simulink model "dcmtr_cl_init"  (R2024a)
settings: Solver=ode15s  StartTime=0.0  StopTime=10  RelTol=1e-3
PostLoadFcn:
  | load('dcmtr_params.mat');
libraries: slpidlib x1
settings Model: Creator=smuckati  LastModifiedBy=smuckati
settings DebuggingCC: ParameterPrecisionLossMsg=none  UnconnectedInputMsg=warning  UnconnectedOutputMsg=warning  UnconnectedLineMsg=warning
settings ModelReferenceCC: EnableRefExpFcnMdlSchedulingChecks=on
settings RTWCC: GPUComputeCapability=3.5  DLArmComputeVersion=19.05

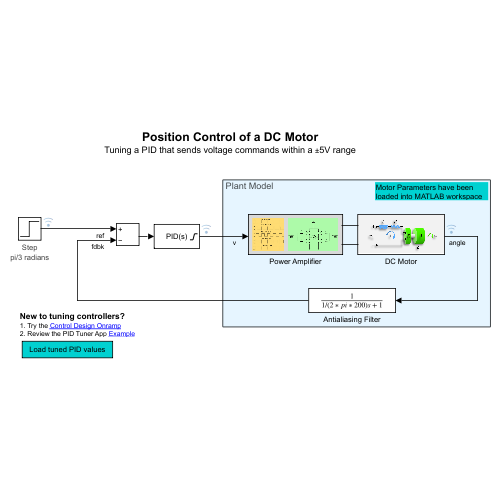
[thumbnail: Simulink's stored preview of the top-level diagram]
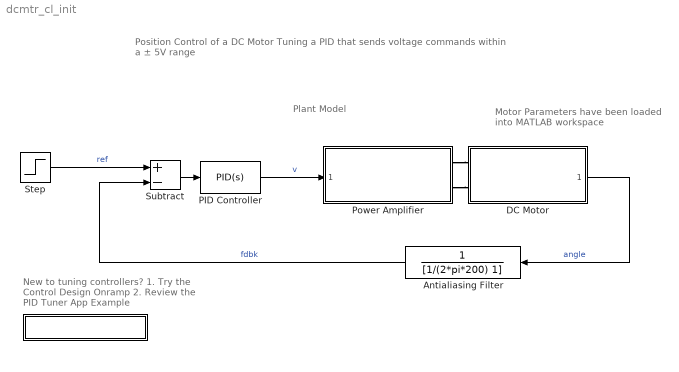
== system dcmtr_cl_init ==
  note: Motor Parameters have been loaded into MATLAB workspace
  note: Position Control of a DC Motor
      | Tuning a PID that sends voltage commands within a ± 5V range
  note: Plant Model
  note: New to tuning controllers?
      | 1. Try the Control Design Onramp
      | 2. Review the PID Tuner App Example
  "   " : Subsystem
      settings: OpenFcn=|
      | load('dcmtr_params.mat')
      | PVal = get_param('dcmtr_cl_init/PID Controller', 'P');
      | 
      | if str2num(PVal) == 1
      | set_param('dcmtr_cl_init/PID Controller', 'P', '80')
      | set_param('dcmtr_cl_init/PID Controller', 'I', '60')
      | set_param('dcmtr_cl_init/PID Controller', 'D', '-2.214')
      | set_param('dcmtr_cl_init/PID Controller', 'N', '7')
      | set_param(gcs,'SimulationCommand','update');
      | msgbox('Tuned parameters loaded to PID block')
      | end
      | 
      | if str2num(PVal) == 80
      | set_param('dcmtr_cl_init/PID Controller', 'P', '1')
      | set_param('dcmtr_cl_init/PID Controller', 'I', '1')
      | set_param('dcmtr_cl_init/PID Controller', 'D', '0')
      | set_param('dcmtr_cl_init/PID Controller', 'N', '100')
      | set_param(gcs,'SimulationCommand','update');
      | msgbox('Initial parameter values loaded to PID Block')
      | end
      mask Display:
      | PVal = get_param('dcmtr_cl_init/PID Controller', 'P');
      | 
      | if str2num(PVal) == 80
      | disp('Load initial PID values')
      | end
      | 
      | if str2num(PVal) == 1
      | disp('Load tuned PID values')
      | end
  Antialiasing Filter : TransferFcn  Denominator=[1/(2*pi*200) 1]
  DC Motor : Subsystem  ReferencedSubsystem=dcmtr
  PID Controller : slpidlib/PID Controller  Controller=PID  Form=Parallel  TimeDomain=Continuous-time  UseExternalTs=off  SampleTime=-1  IntegratorMethod=Forward Euler  FilterMethod=Forward Euler  ControllerParametersSource=internal  P=1  I=1  UseKiTs=off  D=0  UseExternalDerivativeSource=off  N=100  UseFilter=on  TunerSelectOption=Transfer Function Based (PID Tuner App)  InitialConditionSource=internal  InitialConditionForIntegrator=0  InitialConditionForFilter=0  DifferentiatorICPrevScaledInput=0  ExternalReset=none  TrackingMode=off  Kt=1  LimitOutput=on  SatLimitsSource=internal  UpperSaturationLimit=5  LowerSaturationLimit=-5  LinearizeAsGain=on  AntiWindupMode=none  Kb=1  LimitIntegrator=off  UpperIntegratorSaturationLimit=inf  LowerIntegratorSaturationLimit=-inf  POutMin=[]  POutMax=[]  IOutMin=[]  IOutMax=[]  DOutMin=[]  DOutMax=[]  NOutMin=[]  NOutMax=[]  SumOutMin=[]  SumOutMax=[]  SaturationOutMin=[]  SaturationOutMax=[]  PParamMin=[]  PParamMax=[]  IParamMin=[]  IParamMax=[]  DParamMin=[]  DParamMax=[]  NParamMin=[]  NParamMax=[]  KbParamMin=[]  KbParamMax=[]  KtParamMin=[]  KtParamMax=[]  KbOutMin=[]  KbOutMax=[]  KtOutMin=[]  KtOutMax=[]  IntegratorOutMin=[]  IntegratorOutMax=[]  FilterOutMin=[]  FilterOutMax=[]  SumI1OutMin=[]  SumI1OutMax=[]  SumI2OutMin=[]  SumI2OutMax=[]  SumI3OutMin=[]  SumI3OutMax=[]  SumI4OutMin=[]  SumI4OutMax=[]  SumDOutMin=[]  SumDOutMax=[]  DifferentiatorOutMin=[]  DifferentiatorOutMax=[]  FilterDiffOutCoefMin=[]  FilterDiffOutCoefMax=[]  ReciprocalOutMin=[]  ReciprocalOutMax=[]  SumDenOutMin=[]  SumDenOutMax=[]  SumNumOutMin=[]  SumNumOutMax=[]  DivideOutMin=[]  DivideOutMax=[]  UdiffTsProdOutMin=[]  UdiffTsProdOutMax=[]  NTsProdOutMin=[]  NTsProdOutMax=[]  UintegralTsProdOutMin=[]  UintegralTsProdOutMax=[]  UngainTsProdOutMin=[]  UngainTsProdOutMax=[]  ClampingZeroOutDataTypeStr=Inherit: Inherit via back propagation  ClampingZeroOutMin=[]  ClampingZeroOutMax=[]  FilterDenConstantOutDataTypeStr=Inherit: Inherit via back propagation  FilterDenConstantOutMin=[]  FilterDenConstantOutMax=[]  PCopyOutDataTypeStr=Inherit: Inherit via back propagation  PCopyOutMin=[]  PCopyOutMax=[]  NCopyOutDataTypeStr=Inherit: Inherit via back propagation  NCopyOutMin=[]  NCopyOutMax=[]  IntegratorContinuousStateAttributes=''  IntegratorStateMustResolveToSignalObject=off  IntegratorRTWStateStorageClass=Auto  FilterContinuousStateAttributes=''  FilterStateMustResolveToSignalObject=off  FilterRTWStateStorageClass=Auto  ParallelPVariant=InternalParameters  IdealPVariant=Disabled  IVariant=InternalParameters  DVariant=InternalParameters  IntegratorVariant=Continuous  SatVariant=Enabled  AWVariant=Passthrough  PCopyVariant=Disabled  TRVariant=Disabled  FdbkBlocksVariant=Forward  IdealPFdbkVariant=Disabled  SatFdbkVariant=Disabled  DerivativeFilterVariant=ContFilter  NVariant=InternalParameters  NCopyVariant=Disabled  FilterICVariant=InternalICsFilter  IntegratorICVariant=InternalICs  ExternalResetVariant=Disabled  TRSumVariant=Passthrough  SumFdbkVariant=Disabled  SumVariant=Sum_PID  TsampFilterVariant=InternalTs  TsampNgainVariant=Passthrough  TsampIntegralVariant=Disabled_SignalSpec  ExternalSaturationOutDataTypeStr=Inherit: Same as second input  DerivativeSourceVariant=ErrorSignal
  Power Amplifier : Subsystem  ReferencedSubsystem=powerAmp
  Step : Step  Time=0  After=pi/3  SampleTime=0
      settings: AttributesFormatString=|
      | %<Name>
      | %<After> radians
  Subtract : Sum  Inputs=+-
  wires:
  Subtract/1 -> PID Controller/1
  DC Motor/1 -> Antialiasing Filter/1  "angle"
  Step/1 -> Subtract/1  "ref"
  Antialiasing Filter/1 -> Subtract/2  "fdbk"
  PID Controller/1 -> Power Amplifier/1  "v"
  connections:
  Power Amplifier/RConn1 -- DC Motor/LConn1
  Power Amplifier/RConn2 -- DC Motor/LConn2

== system dcmtr_cl_init/    ==
